simulink model "corangbuoc"  (R2018b)
settings: Solver=FixedStepAuto  StartTime=0.0  StopTime=10.0  FixedStep=0.001  RelTol=1e-3
settings Model: Creator=User  LastModifiedBy=User

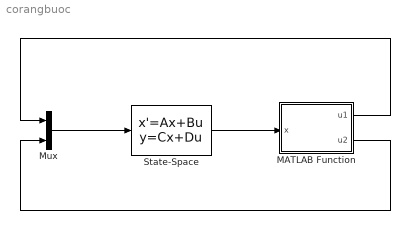
== system corangbuoc ==
  MATLAB Function : MATLAB Function  TreatAsAtomicUnit=on
  Mux : Mux  Inputs=2
  State-Space : StateSpace  A=[2 1 1;1 -1 0;0 0 1]  B=[0 0;0 1;1 0]  C=eye(3)  D=[0 0;0 0;0 0]  InitialCondition=[1;1;1]
  wires:
  State-Space/1 -> MATLAB Function/1(x)
  Mux/1 -> State-Space/1
  MATLAB Function/1(u1) -> Mux/1
  MATLAB Function/2(u2) -> Mux/2

== matlab function corangbuoc/MATLAB Function ==
  data: x input; u1 output; u2 output
function [u1,u2] = fcn(x)
u1=-tanh(1/3*(7.8826*x(1)+2.3814*x(2)+4.6328*x(3)+3.2928*x(1)^3+2.7922*x(1)^2*x(2)+4.4431*x(1)*x(2)*x(3)+0.8222*x(1)*x(2)^2+7.4536*x(1)^2*x(3)+5.8834*x(1)*x(3)^2+0.0862*x(2)^3+0.6420*x(2)^2*x(3)+1.7905*x(2)*x(3)^2+1.6398*x(3)^3))*3;
u2=-tanh(1/20*(9.4324*x(1)+2.8903*x(2)+2.3814*x(3)-0.0647*x(1)^3+0.0842*x(1)^2*x(2)+1.6443*x(1)*x(2)*x(3)+0.1226*x(1)*x(2)^2+2.7922*x(1)^2*x(3)+2.2215*x(1)*x(3)^2+0.0158*x(2)^3+0.2585*x(2)^2*x(3)+0.642*x(2)*x(3)^2+0.5968*x(3)^3))*20;
